simulink model "VCO_DSM_dual_05"  (R2020b)
settings: Solver=VariableStepAuto  StartTime=0.0  StopTime=230*152e-9  RelTol=1e-3
model workspace (MAT data in the model file):
  KVCO_C = 84300000
values from neighbouring files (symbols this model uses):
  clk_p = 1/clk    (= 5e-09)    [parallel_simulink_test8.m]
  finw = 2*pi*M/(N_in*clk_p)    (= 3374757.73335)    [parallel_simulink_test8.m]
  Ph2 = circshift(Ph, (N_stage+1)/2)    [parallel_simulink_test8.m]
undefined symbols (not defined in the file or in its folder): Amp_in, Bias, Compen, fc_fixed, fit_curve, gain_DAC, kvco_fixed, Ph
libraries: commblksprivate x4, simulink_extras x3, dspsigattribs x2, commsynccomp2 x2, simulink x1
settings Model: Creator=97826  LastModifiedBy=97826

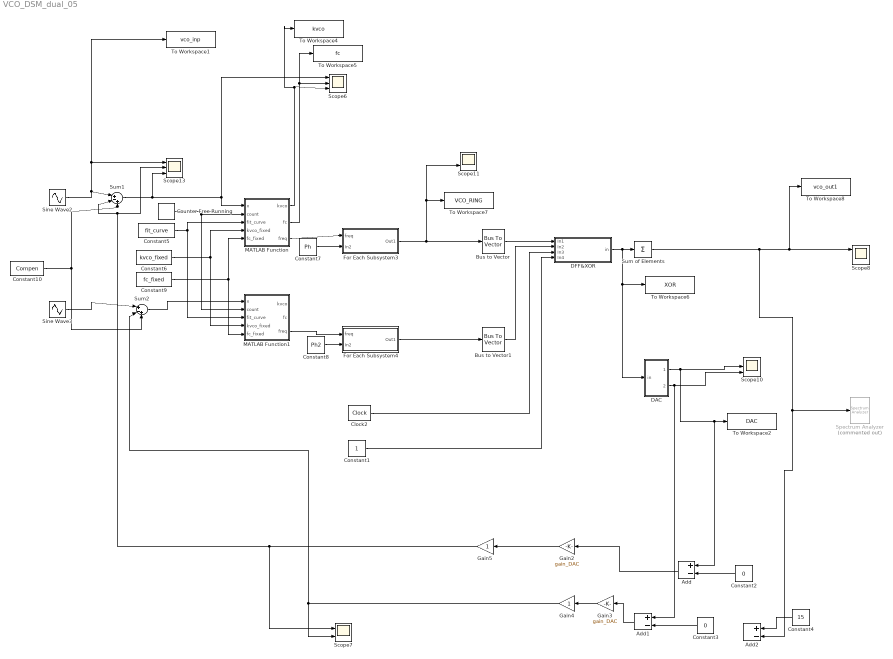
== system VCO_DSM_dual_05 ==
  Add : Sum  Inputs=+-
  Add1 : Sum  Inputs=+-
  Add2 : Sum  Inputs=+-
  Bus to Vector : BusToVector
  Bus to Vector1 : BusToVector
  Clock2 : simulink_extras/Flip Flops/Clock  period=clk_p
  Constant1 : Constant
  Constant10 : Constant  Value=Compen
  Constant2 : Constant  Value=0
  Constant3 : Constant  Value=0
  Constant4 : Constant  Value=15
  Constant5 : Constant  Value=fit_curve  VectorParams1D=off
  Constant6 : Constant  Value=kvco_fixed  VectorParams1D=off
  Constant7 : Constant  Value=Ph  VectorParams1D=off
  Constant8 : Constant  Value=Ph2  VectorParams1D=off
  Constant9 : Constant  Value=fc_fixed  VectorParams1D=off
  Counter Free-Running : simulink/Sources/Counter Free-Running  NumBits=32  tsamp=clk_p
  DAC : Subsystem
  DFF&XOR : Subsystem  TreatAsAtomicUnit=on
  For Each Subsystem3 : Subsystem  TreatAsAtomicUnit=on
  For Each Subsystem4 : Subsystem  TreatAsAtomicUnit=on
  Gain2 : Gain  Gain=gain_DAC
  Gain3 : Gain  Gain=gain_DAC
  Gain4 : Gain
  Gain5 : Gain
  MATLAB Function : MATLAB Function  TreatAsAtomicUnit=on
  MATLAB Function1 : MATLAB Function  TreatAsAtomicUnit=on
  Scope{6,8,10,13} (4 alike) : Scope  NumInputPorts=3
  Scope11 : Scope  NumInputPorts=2
  Scope7 : Scope  NumInputPorts=2
  Sine Wave2 : Sin  Amplitude=Amp_in  Bias=Bias  Frequency=finw  SampleTime=0
  Sine Wave3 : Sin  Amplitude=Amp_in  Bias=Bias  Frequency=finw  Phase=pi  SampleTime=0
  Spectrum Analyzer : SpectrumAnalyzer  Commented=on
  Sum of Elements : Sum  Inputs=+  CollapseMode=Specified dimension
  Sum1 : Sum  Inputs=|+-+
  Sum2 : Sum  Inputs=|+-+
  To Workspace1 : ToWorkspace  VariableName=vco_inp  SampleTime=-1
  To Workspace2 : ToWorkspace  VariableName=DAC  SampleTime=-1
  To Workspace4 : ToWorkspace  VariableName=kvco  SampleTime=-1
  To Workspace5 : ToWorkspace  VariableName=fc  SampleTime=-1
  To Workspace6 : ToWorkspace  VariableName=XOR  SampleTime=-1
  To Workspace7 : ToWorkspace  VariableName=VCO_RING  SampleTime=-1
  To Workspace8 : ToWorkspace  VariableName=vco_out1  SampleTime=-1
  wires:
  Sum2/1 -> MATLAB Function1/1(x)
  Gain5/1 -> Scope13/2, Sum1/2, Scope7/1
  Sine Wave2/1 -> Scope13/1, To Workspace1/1, Sum1/1
  Gain4/1 -> Scope7/2, Sum2/2
  Gain3/1 -> Gain4/1
  Sine Wave3/1 -> Sum2/1
  Gain2/1 -> Gain5/1
  Clock2/1 -> DFF&XOR/3(In3)
  Constant1/1 -> DFF&XOR/4(In4)
  Sum1/1 -> Scope13/3, Scope6/1, MATLAB Function/1(x)
  Constant2/1 -> Add/2
  Constant3/1 -> Add1/2
  Add1/1 -> Gain3/1
  Add/1 -> Gain2/1
  MATLAB Function/1(kvco) -> Scope6/3, To Workspace4/1
  MATLAB Function/2(fc) -> Scope6/2, To Workspace5/1
  MATLAB Function/3(freq) -> For Each Subsystem3/1(freq)
  MATLAB Function1/3(freq) -> For Each Subsystem4/1(freq)
  Bus to Vector/1 -> DFF&XOR/1(In1)
  Bus to Vector1/1 -> DFF&XOR/2(In2)
  DFF&XOR/1(in) -> To Workspace6/1, DAC/1(in), Sum of Elements/1
  DAC/1(out1) -> Add/1, To Workspace2/1, Scope10/2
  DAC/2(out2) -> Add1/1, Scope10/3
  Constant4/1 -> Add2/1
  Sum of Elements/1 -> Spectrum Analyzer/1, Add2/2, Scope8/1, To Workspace8/1
  Counter Free-Running/1 -> MATLAB Function1/2(count), MATLAB Function/2(count)
  Constant7/1 -> For Each Subsystem3/2(In2)
  For Each Subsystem3/1(Out1) -> To Workspace7/1, Scope11/2, Bus to Vector/1
  Constant8/1 -> For Each Subsystem4/2(In2)
  For Each Subsystem4/1(Out1) -> Bus to Vector1/1
  Constant5/1 -> MATLAB Function1/3(fit_curve), MATLAB Function/3(fit_curve)
  Constant6/1 -> MATLAB Function1/4(kvco_fixed), MATLAB Function/4(kvco_fixed)
  Constant9/1 -> MATLAB Function/5(fc_fixed), MATLAB Function1/5(fc_fixed)
  Constant10/1 -> Sum1/3, Sum2/3

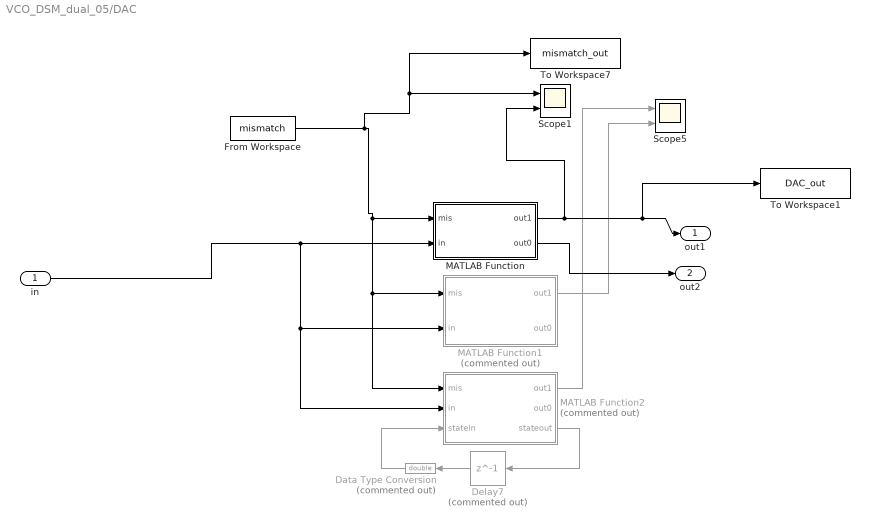
== system VCO_DSM_dual_05/DAC ==
  in : Inport
  Data Type Conversion : DataTypeConversion  Commented=on  OutDataTypeStr=double
  Delay7 : Delay  Commented=on  DelayLength=1  SampleTime=clk_p
  From Workspace : FromWorkspace  VariableName=mismatch
  MATLAB Function : MATLAB Function  TreatAsAtomicUnit=on
  MATLAB Function1 : MATLAB Function  Commented=on  TreatAsAtomicUnit=on
  MATLAB Function2 : MATLAB Function  Commented=on  TreatAsAtomicUnit=on
  Scope1 : Scope  NumInputPorts=2
  Scope5 : Scope  NumInputPorts=2
  To Workspace1 : ToWorkspace  VariableName=DAC_out  SampleTime=-1
  To Workspace7 : ToWorkspace  VariableName=mismatch_out  SampleTime=-1
  out1 : Outport
  out2 : Outport  Port=2
  wires:
  From Workspace/1 -> To Workspace7/1, Scope1/1, MATLAB Function2/1(mis), MATLAB Function1/1(mis), MATLAB Function/1(mis)
  MATLAB Function1/1(out1) -> Scope5/2
  MATLAB Function2/1(out1) -> Scope5/1
  MATLAB Function2/3(stateout) -> Delay7/1
  Delay7/1 -> Data Type Conversion/1
  Data Type Conversion/1 -> MATLAB Function2/3(statein)
  MATLAB Function/1(out1) -> Scope1/2, To Workspace1/1, out1/1
  MATLAB Function/2(out0) -> out2/1
  in/1 -> MATLAB Function2/2(in), MATLAB Function1/2(in), MATLAB Function/2(in)

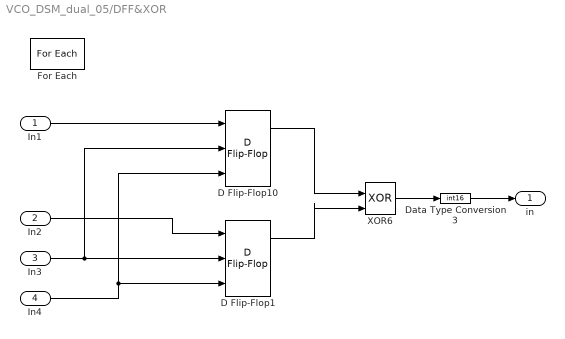
== system VCO_DSM_dual_05/DFF&XOR ==
  In1 : Inport  Partition=on  PartitionDimension=1  PartitionWidth=N_stage  PartitionOffset=0
  In2 : Inport  Port=2  Partition=on  PartitionDimension=1  PartitionWidth=N_stage  PartitionOffset=0
  In3 : Inport  Port=3
  In4 : Inport  Port=4
  D Flip-Flop1 : simulink_extras/Flip Flops/D Flip-Flop
  D Flip-Flop10 : simulink_extras/Flip Flops/D Flip-Flop
  Data Type Conversion3 : DataTypeConversion  OutDataTypeStr=int16
  For Each : ForEach  DisableCoverage=on
  XOR6 : Logic  Operator=XOR  IconShape=distinctive  AllPortsSameDT=off  OutDataTypeStr=boolean
  in : Outport  ConcatenationDimension=1
  wires:
  In1/1 -> D Flip-Flop10/1
  In3/1 -> D Flip-Flop1/2, D Flip-Flop10/2
  In4/1 -> D Flip-Flop1/3, D Flip-Flop10/3
  In2/1 -> D Flip-Flop1/1
  D Flip-Flop10/1 -> XOR6/1
  D Flip-Flop1/1 -> XOR6/2
  XOR6/1 -> Data Type Conversion3/1
  Data Type Conversion3/1 -> in/1

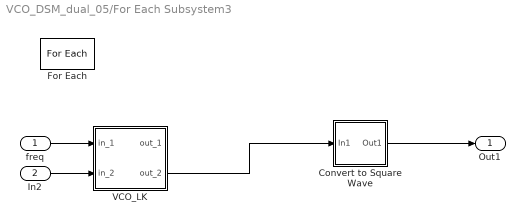
== system VCO_DSM_dual_05/For Each Subsystem3 ==
  freq : Inport
  In2 : Inport  Port=2  Partition=on  PartitionDimension=1  PartitionWidth=1  PartitionOffset=0
  Convert to Square Wave : Subsystem
  For Each : ForEach  DisableCoverage=on
  VCO_LK : Subsystem  mask{Ac=1, Fc=1, Kc=1, Ph=1}
  Out1 : Outport  ConcatenationDimension=1
  wires:
  freq/1 -> VCO_LK/1(in_1)
  Convert to Square Wave/1(Out1) -> Out1/1
  VCO_LK/2(out_2) -> Convert to Square Wave/1(In1)
  In2/1 -> VCO_LK/2(in_2)

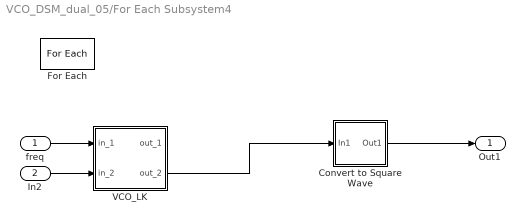
== system VCO_DSM_dual_05/For Each Subsystem4 ==
  freq : Inport
  In2 : Inport  Port=2  Partition=on  PartitionDimension=1  PartitionWidth=1  PartitionOffset=0
  Convert to Square Wave : Subsystem
  For Each : ForEach  DisableCoverage=on
  VCO_LK : Subsystem  mask{Ac=1, Fc=1, Kc=1, Ph=1}
  Out1 : Outport  ConcatenationDimension=1
  wires:
  freq/1 -> VCO_LK/1(in_1)
  Convert to Square Wave/1(Out1) -> Out1/1
  VCO_LK/2(out_2) -> Convert to Square Wave/1(In1)
  In2/1 -> VCO_LK/2(in_2)

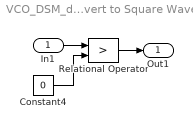
== system VCO_DSM_dual_05/For Each Subsystem3/Convert to Square Wave ==
  In1 : Inport
  Constant4 : Constant  Value=0
  Relational Operator : RelationalOperator  Operator=>  RndMeth=Nearest  InputSameDT=on
  Out1 : Outport
  wires:
  Relational Operator/1 -> Out1/1
  In1/1 -> Relational Operator/1
  Constant4/1 -> Relational Operator/2

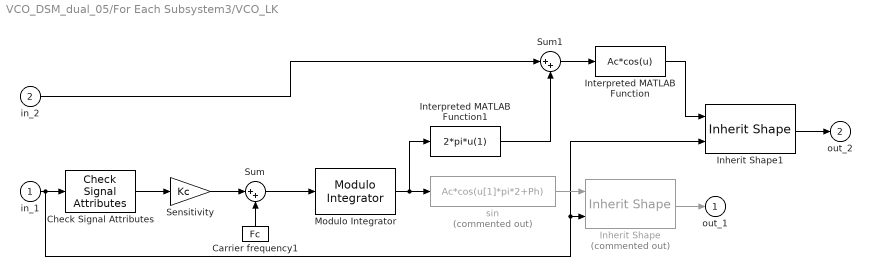
== system VCO_DSM_dual_05/For Each Subsystem3/VCO_LK ==
  in_1 : Inport
  in_2 : Inport  Port=2
  Carrier frequency1 : Constant  Value=Fc
  Check Signal Attributes : dspsigattribs/Check Signal Attributes  SigAttribCheckMethod=Does not match attributes exactly  Complexity=Ignore  Frame=Sample-based  DimsCheckMethod=Ignore  Dimensions=Vector (1-D or 2-D) or scalar  DatatypeCheckMethod=Ignore  DatatypeGeneral=Floating-point  DtypeFloatSpecific=Double precision  DtypeFixedSpecific=Any fixed-point  DtypeIntSpecific=Any integer  SampleMode=Ignore
      settings: SourceProductName=DSP System Toolbox
  Inherit Shape : commblksprivate/Inherit Shape  Commented=on
      settings: SourceProductBaseCode=CM
  Inherit Shape1 : commblksprivate/Inherit Shape
      settings: SourceProductBaseCode=CM
  Interpreted MATLAB Function : MATLABFcn  MATLABFcn=Ac*cos(u)
  Interpreted MATLAB Function1 : MATLABFcn  MATLABFcn=2*pi*u(1)
  Modulo Integrator : commsynccomp2/Continuous-Time VCO/Modulo  Integrator  SystemSampleTime=-1  VariantActivationTime=update diagram  Latency=0  AutoFrameSizeCalculation=off
      settings: SourceProductBaseCode=CM
  Sensitivity : Gain  Gain=Kc  SaturateOnIntegerOverflow=on  OutDataTypeStr=Inherit: Same as input  ParamDataTypeStr=Inherit: Same as input
  Sum : Sum  Inputs=|++  InputSameDT=on  SaturateOnIntegerOverflow=on  OutDataTypeStr=Inherit: Same as first input
  Sum1 : Sum  Inputs=|++  InputSameDT=on  SaturateOnIntegerOverflow=on  OutDataTypeStr=Inherit: Same as first input
  sin : Fcn  Commented=on  Expr=Ac*cos(u[1]*pi*2+Ph)
  out_1 : Outport  InitialOutput=0  VectorParamsAs1DForOutWhenUnconnected=off
  out_2 : Outport  Port=2  InitialOutput=0  VectorParamsAs1DForOutWhenUnconnected=off
  wires:
  Sum/1 -> Modulo Integrator/1
  Modulo Integrator/1 -> Interpreted MATLAB Function1/1, sin/1
  Carrier frequency1/1 -> Sum/2
  Inherit Shape/1 -> out_1/1
  Check Signal Attributes/1 -> Sensitivity/1
  in_1/1 -> Check Signal Attributes/1, Inherit Shape1/2, Inherit Shape/2
  sin/1 -> Inherit Shape/1
  Sensitivity/1 -> Sum/1
  in_2/1 -> Sum1/1
  Sum1/1 -> Interpreted MATLAB Function/1
  Interpreted MATLAB Function1/1 -> Sum1/2
  Interpreted MATLAB Function/1 -> Inherit Shape1/1
  Inherit Shape1/1 -> out_2/1

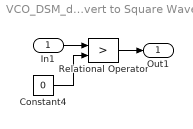
== system VCO_DSM_dual_05/For Each Subsystem4/Convert to Square Wave ==
  In1 : Inport
  Constant4 : Constant  Value=0
  Relational Operator : RelationalOperator  Operator=>  RndMeth=Nearest  InputSameDT=on
  Out1 : Outport
  wires:
  Relational Operator/1 -> Out1/1
  In1/1 -> Relational Operator/1
  Constant4/1 -> Relational Operator/2

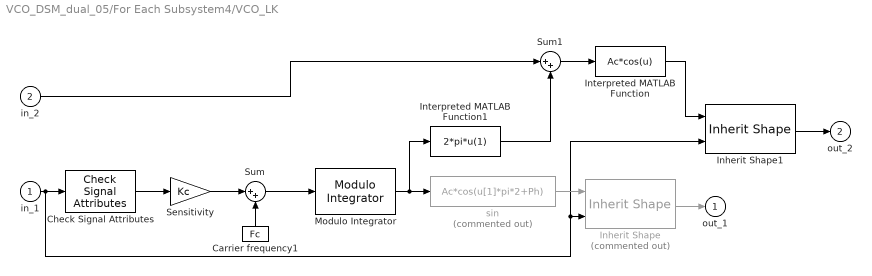
== system VCO_DSM_dual_05/For Each Subsystem4/VCO_LK ==
  in_1 : Inport
  in_2 : Inport  Port=2
  Carrier frequency1 : Constant  Value=Fc
  Check Signal Attributes : dspsigattribs/Check Signal Attributes  SigAttribCheckMethod=Does not match attributes exactly  Complexity=Ignore  Frame=Sample-based  DimsCheckMethod=Ignore  Dimensions=Vector (1-D or 2-D) or scalar  DatatypeCheckMethod=Ignore  DatatypeGeneral=Floating-point  DtypeFloatSpecific=Double precision  DtypeFixedSpecific=Any fixed-point  DtypeIntSpecific=Any integer  SampleMode=Ignore
      settings: SourceProductName=DSP System Toolbox
  Inherit Shape : commblksprivate/Inherit Shape  Commented=on
      settings: SourceProductBaseCode=CM
  Inherit Shape1 : commblksprivate/Inherit Shape
      settings: SourceProductBaseCode=CM
  Interpreted MATLAB Function : MATLABFcn  MATLABFcn=Ac*cos(u)
  Interpreted MATLAB Function1 : MATLABFcn  MATLABFcn=2*pi*u(1)
  Modulo Integrator : commsynccomp2/Continuous-Time VCO/Modulo  Integrator  SystemSampleTime=-1  VariantActivationTime=update diagram  Latency=0  AutoFrameSizeCalculation=off
      settings: SourceProductBaseCode=CM
  Sensitivity : Gain  Gain=Kc  SaturateOnIntegerOverflow=on  OutDataTypeStr=Inherit: Same as input  ParamDataTypeStr=Inherit: Same as input
  Sum : Sum  Inputs=|++  InputSameDT=on  SaturateOnIntegerOverflow=on  OutDataTypeStr=Inherit: Same as first input
  Sum1 : Sum  Inputs=|++  InputSameDT=on  SaturateOnIntegerOverflow=on  OutDataTypeStr=Inherit: Same as first input
  sin : Fcn  Commented=on  Expr=Ac*cos(u[1]*pi*2+Ph)
  out_1 : Outport  InitialOutput=0  VectorParamsAs1DForOutWhenUnconnected=off
  out_2 : Outport  Port=2  InitialOutput=0  VectorParamsAs1DForOutWhenUnconnected=off
  wires:
  Sum/1 -> Modulo Integrator/1
  Modulo Integrator/1 -> Interpreted MATLAB Function1/1, sin/1
  Carrier frequency1/1 -> Sum/2
  Inherit Shape/1 -> out_1/1
  Check Signal Attributes/1 -> Sensitivity/1
  in_1/1 -> Check Signal Attributes/1, Inherit Shape1/2, Inherit Shape/2
  sin/1 -> Inherit Shape/1
  Sensitivity/1 -> Sum/1
  in_2/1 -> Sum1/1
  Sum1/1 -> Interpreted MATLAB Function/1
  Interpreted MATLAB Function1/1 -> Sum1/2
  Interpreted MATLAB Function/1 -> Inherit Shape1/1
  Inherit Shape1/1 -> out_2/1

== matlab function VCO_DSM_dual_05/MATLAB Function ==
  data: x input; kvco output; fc output; freq output; count input; fit_curve input; kvco_fixed input; fc_fixed input
function [kvco, fc, freq]= f_fit(x,count,fit_curve,kvco_fixed, fc_fixed)
popt = [ 4.13440e+01,  1.83172e+01,  5.20871e+00];
%[ 3.77235e+01,  1.83291e+01,  5.29554e+00]% 5mV step fitting curve
a = popt(1);
b = popt(2);
c = popt(3);
%fc = 737e3;%a * exp(b * x + c);
if (fit_curve)
    if (count>500) % 0.2 ensure is stable %x<-100 %(false)%
        if(x>0.35)
            fc = 4.6e6;
            kvco = 84.3e6;
        else
        fc = a * exp(b * x + c);
        kvco = 138478.796252113*exp(18.3171808515013*x);
        %kvco_5mV = 137904.821055187*exp(18.3291161903355*x); % 5mV step fitting curve
        end
    else
        fc = 4.6e6;%737e3;%a * exp(b * x + c);
        kvco = 84.3e6;%30e6;%138478.796252113*exp(18.3171808515013*x);
    end
else
    fc = fc_fixed;%4.6e6;%737e3;%a * exp(b * x + c);
    kvco = kvco_fixed;%84.3e6;  
end

freq = kvco*x + fc;
end

== matlab function VCO_DSM_dual_05/MATLAB Function1 ==
  data: x input; kvco output; fc output; freq output; count input; fit_curve input; kvco_fixed input; fc_fixed input
function [kvco, fc, freq]= f_fit(x,count,fit_curve,kvco_fixed, fc_fixed)
popt = [ 4.13440e+01,  1.83172e+01,  5.20871e+00];
a = popt(1);
b = popt(2);
c = popt(3);
%fc = 737e3;%a * exp(b * x + c);
if (fit_curve)
    if (count>500) % 0.2 ensure is stable %x<-100 %(false)%
        if(x>0.35)%>0.35
            fc = 4.6e6;
            kvco = 84.3e6;
        else
        fc = a * exp(b * x + c);
        kvco = 138478.796252113*exp(18.3171808515013*x);
        end
    else
        fc = 4.6e6;%737e3;%a * exp(b * x + c);
        kvco = 84.3e6;%30e6;%138478.796252113*exp(18.3171808515013*x);
    end
else
    fc = fc_fixed;%4.6e6;%737e3;%a * exp(b * x + c);
    kvco = kvco_fixed;%84.3e6;  
end

freq = kvco*x + fc;
end

== matlab function VCO_DSM_dual_05/DAC/MATLAB Function ==
  data: mis input; out1 output; in input; out0 output
function [out1, out0]= DAC_CLA(mis, in)
out1 = 0;
out0 = 0;
b = size(mis);
t = b(1);
for i = 1:t %15
    if (in(i)==1)
        out1 = out1 + mis(i);
    else
        out0 = out0 + mis(i);
    end
end
end

== matlab function VCO_DSM_dual_05/DAC/MATLAB Function1 ==
  data: mis input; out1 output; in input; out0 output
function [out1, out0]= DAC_thermo(mis, in)
out1 = 0;
out0 = 0;
sum = int16(0);
sum_mis = 0;

for i = 1:15
    sum = sum + in(i);
    sum_mis= sum_mis + mis(i);
end

for j = 1:sum
    out1 = out1 + mis(j);
end

out0 = sum_mis - out1;
end

== matlab function VCO_DSM_dual_05/DAC/MATLAB Function2 ==
  data: mis input; out1 output; in input; out0 output; statein input; stateout output
function [out1, out0, stateout]= DAC_DWA(mis, in,statein)
enable = 1;
out1 = 0;
out0 = 0;
data = int16(0);

bitout=zeros(15,1);

for i = 1:15
    data = data + in(i);
end


stateplus=data;
if enable==0;
    stateout=statein;
else
    stateout=statein+stateplus;
end

if (stateout>14)
    stateout=stateout-15;
end

for i=15:-1:1
    if (stateout+data<15)
        if (i<stateout+1 || i>(stateout+data))
        bitout(i)=0;
        else
            bitout(i)=1;
        end
    else
        if (i>stateout || i<(stateout+data-14))
        bitout(i)=1;
        else
            bitout(i)=0;
        end
    end
end

for i = 1:15
    if (bitout(i)==1)
        out1 = out1 + mis(i);
    else
        out0 = out0 + mis(i);
    end
end

end
